simulink model "simuleGearogMotor"  (Simulink 7.4)
settings: Solver=ode45  StartTime=0.0  StopTime=80.0  RelTol=1e-3
values from neighbouring files (symbols this model uses):
  Bs = 1.748817703686052e-04    (= 0.000174881770369)    [verifikationgear.m]
  Js = 2.686970843428432e-04    (= 0.000268697084343)    [verifikationgear.m]
  Km = 0.022141706562986    (= 0.022141706563)    [verifikationgear.m]
  Rm = 0.807790757873553    (= 0.807790757874)    [verifikationgear.m]
settings Model: Creator=Skov  LastModifiedBy=Skov

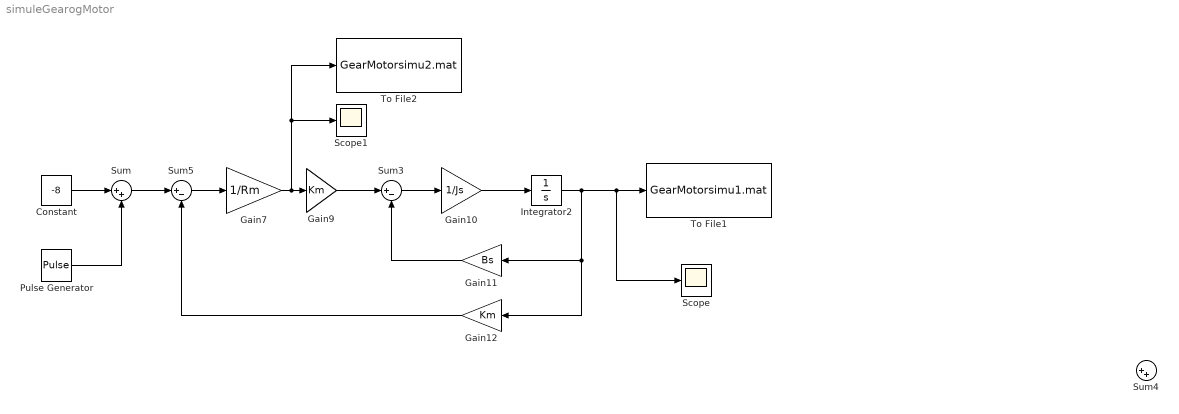
== system simuleGearogMotor ==
  Constant : Constant  Value=-8  OutDataType=fixdt(1, 16)  OutScaling=2^0
  Gain10 : Gain  Gain=1/Js  ParameterDataType=fixdt(1, 16)  ParameterScaling=2^0  OutDataType=fixdt(1, 16)  OutScaling=2^0
  Gain11 : Gain  Gain=Bs  ParameterDataType=fixdt(1, 16)  ParameterScaling=2^0  OutDataType=fixdt(1, 16)  OutScaling=2^0
  Gain12 : Gain  Gain=Km  ParameterDataType=fixdt(1, 16)  ParameterScaling=2^0  OutDataType=fixdt(1, 16)  OutScaling=2^0
  Gain7 : Gain  Gain=1/Rm  ParameterDataType=fixdt(1, 16)  ParameterScaling=2^0  OutDataType=fixdt(1, 16)  OutScaling=2^0
  Gain9 : Gain  Gain=Km  ParameterDataType=fixdt(1, 16)  ParameterScaling=2^0  OutDataType=fixdt(1, 16)  OutScaling=2^0
  Integrator2 : Integrator
  Pulse Generator : DiscretePulseGenerator  PulseType=Time based  Amplitude=16  Period=10  PulseWidth=50  PhaseDelay=0  SampleTime=1
  Scope : Scope
  Scope1 : Scope
  Sum : Sum  Inputs=|++  OutDataType=fixdt(1, 16)  OutScaling=2^0
  Sum3 : Sum  Inputs=|+-  OutDataType=fixdt(1, 16)  OutScaling=2^0
  Sum4 : Sum  Inputs=|++  OutDataType=fixdt(1, 16)  OutScaling=2^0
  Sum5 : Sum  Inputs=|+-  OutDataType=fixdt(1, 16)  OutScaling=2^0
  To File1 : ToFile  Filename=GearMotorsimu1.mat  SampleTime=0.01
  To File2 : ToFile  Filename=GearMotorsimu2.mat  SampleTime=0.01
  wires:
  ? -> Sum4/1
  Pulse Generator/1 -> Sum/2
  Constant/1 -> Sum/1
  Gain7/1 -> Gain9/1, Scope1/1, To File2/1
  Gain10/1 -> Integrator2/1
  Sum3/1 -> Gain10/1
  Integrator2/1 -> Gain11/1, Gain12/1, Scope/1, To File1/1
  Gain12/1 -> Sum5/2
  Gain11/1 -> Sum3/2
  Gain9/1 -> Sum3/1
  Sum/1 -> Sum5/1
  Sum5/1 -> Gain7/1
